simulink model "MPSK_filter"  (R2016b)
settings: Solver=FixedStepDiscrete  StartTime=0.0  StopTime=1000*(1/10E3)  FixedStep=1/10E3  RelTol=1e-3
values from neighbouring files (symbols this model uses):
  N = log2(M)    [Graph.m]
libraries: commdigbbndpm3 x2, commfilt2 x2, commchan3 x1, commrandsrc3 x1
settings Model: Creator=ak22070  LastModifiedBy=ak22070
settings DataIOCC: ExternalInput=[N]  SaveOutput=off  OutputSaveName=Ber

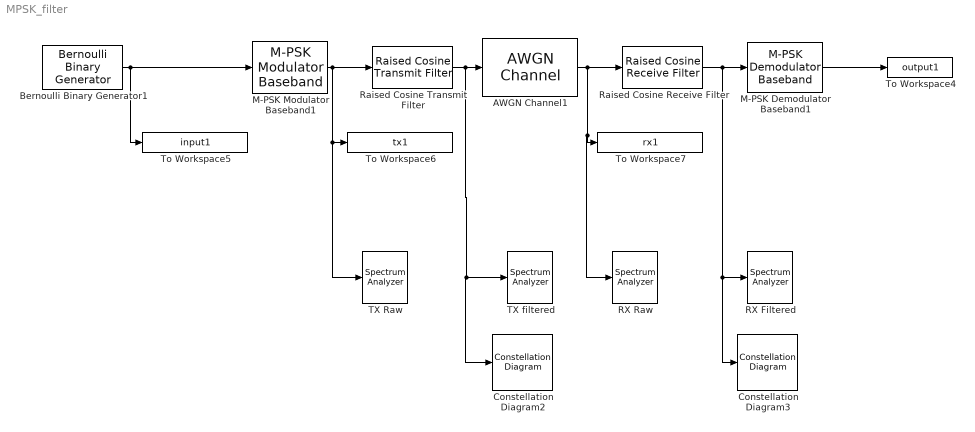
== system MPSK_filter ==
  AWGN Channel1 : commchan3/AWGN Channel  InputProcessing=Columns as channels (frame based)  seed=67  noiseMode="Signal to noise ratio  (Eb/No)"  EbNodB=EbNo  EsNodB=EbNo  SNRdB=10  bitsPerSym=N  Ps=1  Tsym=N  variance=1
  Bernoulli Binary Generator1 : commrandsrc3/Bernoulli Binary Generator  ProbabilityOfZero=0.5  SeedSource=Auto  Seed=0  SampleTime=1  SamplesPerFrame=N*10000  OutputDataType=double  SimulateUsing=Interpreted execution
  Constellation Diagram2 : ConstellationDiagram
  Constellation Diagram3 : ConstellationDiagram
  M-PSK Demodulator Baseband1 : commdigbbndpm3/M-PSK Demodulator Baseband  M=M  OutType=Bit  DecType=Hard decision  VarSource=Dialog  Variance=1  Dec=Gray  Mapping=[0:7]  Ph=pi/8  outDtype1=Inherit via internal rule  outDtype2=double  derotateFactorWordLen=16  derotateFactorDataTypeStr=Inherit: Same word length as input  derotateFactorLastDataTypeStr=Inherit: Same word length as input
  M-PSK Modulator Baseband1 : commdigbbndpm3/M-PSK Modulator Baseband  M=M  InType=Bit  Enc=Gray  Mapping=[0:7]  Ph=pi/8  outDtype=double  outWordLen=16  outUDDataType=sfix(16)  outFracLenMode=Best precision  outFracLen=15  outDataTypeStr=double  outLastDataTypeStr=double
  RX Filtered : SpectrumAnalyzer
  RX Raw : SpectrumAnalyzer
  Raised Cosine Receive Filter : commfilt2/Raised Cosine Receive Filter  filtType=Square root  R=0.33  filtSpan=10  N=N  downFactor=N  downOffset=0  filterGain=1  InputProcessing=Columns as channels (frame based)  RateOptions=Enforce single-rate processing  framing=Mute  checkCoeff=off  variableName=rcRxFilt  currentFiltSpan=10  D=5  inputOffset=0  sampMode=Mute  saveAsFlag=0  rateMode=Downsampling  checkGain=Normalized  launchFVT=on  roundingMode=Floor  overflowMode=off  coeffDataTypeStr=Inherit: Same word length as input  coeffMin=[]  coeffMax=[]  coeffLastDataTypeStr=Inherit: Same word length as input  accumDataTypeStr=Inherit: Same as product output  accumLastDataTypeStr=Inherit: Same as product output  outputDataTypeStr=Inherit: Same as accumulator  outputMin=[]  outputMax=[]  outputLastDataTypeStr=Inherit: Same as accumulator
  Raised Cosine Transmit Filter : commfilt2/Raised Cosine Transmit Filter  filtType=Square root  R=0.33  filtSpan=10  N=N  filterGain=1  InputProcessing=Columns as channels (frame based)  RateOptions=Enforce single-rate processing  framing=Mute  checkCoeff=off  variableName=rcTxFilt  checkGain=Normalized  sampMode=Mute  saveAsFlag=0  currentFiltSpan=10  D=(10)/2  launchFVT=on  roundingMode=Floor  overflowMode=off  coeffDataTypeStr=Inherit: Same word length as input  coeffMin=[]  coeffMax=[]  coeffLastDataTypeStr=Inherit: Same word length as input  outputDataTypeStr=Inherit: Same as accumulator  outputMin=[]  outputMax=[]  outputLastDataTypeStr=Inherit: Same as accumulator
  TX Raw : SpectrumAnalyzer
  TX filtered : SpectrumAnalyzer
  To Workspace4 : ToWorkspace  VariableName=output1  SaveFormat=Timeseries  SampleTime=-1
  To Workspace5 : ToWorkspace  VariableName=input1  SaveFormat=Timeseries  SampleTime=-1
  To Workspace6 : ToWorkspace  VariableName=tx1  SaveFormat=Timeseries  SampleTime=-1
  To Workspace7 : ToWorkspace  VariableName=rx1  SaveFormat=Timeseries  SampleTime=-1
  wires:
  Bernoulli Binary Generator1/1 -> To Workspace5/1, M-PSK Modulator Baseband1/1
  M-PSK Modulator Baseband1/1 -> Raised Cosine Transmit Filter/1, TX Raw/1, To Workspace6/1
  M-PSK Demodulator Baseband1/1 -> To Workspace4/1
  Raised Cosine Transmit Filter/1 -> TX filtered/1, Constellation Diagram2/1, AWGN Channel1/1
  AWGN Channel1/1 -> Raised Cosine Receive Filter/1, RX Raw/1, To Workspace7/1
  Raised Cosine Receive Filter/1 -> Constellation Diagram3/1, RX Filtered/1, M-PSK Demodulator Baseband1/1
